simulink model "time_syn"  (R2016a)
settings: Solver=VariableStepAuto  StartTime=0.0  StopTime=1  RelTol=1e-3
values from neighbouring files (symbols this model uses):
  snr = SNR(i)    [mplot.m]
libraries: commchan3 x2, commdigbbndpm3 x1, commrandsrc2 x1, simulink x1, dspobslib x1, dspxfrm3 x1
settings Model: Creator=dell  LastModifiedBy=dell

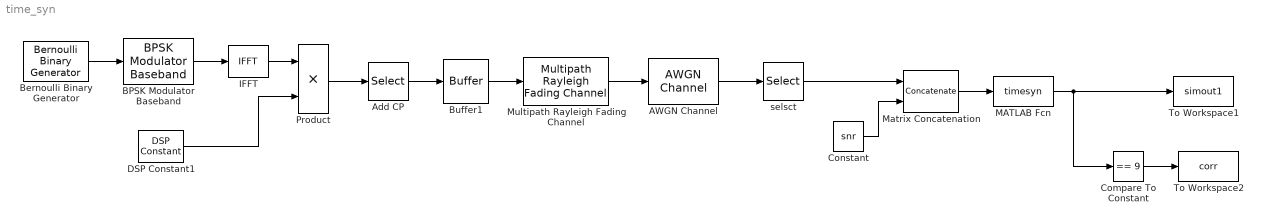
== system time_syn ==
  AWGN Channel : commchan3/AWGN Channel  InputProcessing=Inherited (this choice will be removed - see release notes)  seed=67  noiseMode="Signal to noise ratio  (SNR)"  EbNodB=ebn0  EsNodB=10  SNRdB=snr  bitsPerSym=1  Ps=1  Tsym=1/480000  variance=1
  Add CP : Selector  InputPortWidth=128  IndexOptions=Index vector (dialog)  Indices=[100:128 1:128]  OutputSizes=1
  BPSK Modulator Baseband : commdigbbndpm3/BPSK Modulator Baseband  Ph=0  outDtype=double  outWordLen=16  outUDDataType=sfix(16)  outFracLenMode=Best precision  outFracLen=15  outDataTypeStr=double  outLastDataTypeStr=double
  Bernoulli Binary Generator : commrandsrc2/Bernoulli Binary Generator  P=0.5  seed=565  Ts=1/480000  frameBased=on  sampPerFrame=128  orient=off  outDataType=double
  Buffer1 : Buffer  N=471
  Compare To Constant : simulink/Logic and Bit Operations/Compare To Constant  relop===  const=9  OutDataTypeStr=uint8  ZeroCross=off
  Constant : Constant  Value=snr
  DSP Constant1 : dspobslib/DSP Constant  Value=sqrt(128)  SampleMode=Discrete  discreteOutput=Sample-based  continuousOutput=Sample-based  sampTime=inf  framePeriod=2  dataType=Inherit from 'Constant value'  isSigned=on  wordLen=16  udDataType=sfix(16)  fracBitsMode=Best precision  numFracBits=15  InterpretAs1D=-inf  Ts=-inf  FramebasedOutput=-inf
  IFFT : dspxfrm3/IFFT  FFTImplementation=Auto  CompMethod=Table lookup  TableOpt=HYBRID  TableOptActive=Speed  BitRevOrder=off  cs_in=off  Normalize=on  InheritFFTLength=on  FFTLength=64  WrapInput=on  mode=Complex  outSamplingMode=Frame based  roundingMode=Floor  overflowMode=off  firstCoeffDataTypeStr=Inherit: Same word length as input  firstCoeffLastDataTypeStr=Inherit: Same word length as input  outputMin=[]  outputMax=[]
  MATLAB Fcn : MATLABFcn  MATLABFcn=timesyn  Output1D=off
  Matrix Concatenation : Concatenate  Mode=Multidimensional array
  Multipath Rayleigh Fading Channel : commchan3/Multipath Rayleigh Fading Channel  maxDopplerShift=40  spectrumType=Jakes  sigmaGaussian=1/sqrt(2)  coeffRounded=[1 -1.72 0.785]  freqMinMaxRJakes=[0 1]  freqMinMaxAJakes=[0 1]  sigmaGaussian1=1/sqrt(2)  sigmaGaussian2=1/sqrt(2)  centerFreqGaussian1=0.0  centerFreqGaussian2=0.0  gainGaussian1=0.5  gainGaussian2=0.5  coeffBell=9  dopplerSpectrum=doppler.jakes  pathDelays=[0 ]  avgPathGaindB=[0 ]  normalizePathGains=on  seed=73  enableProbe=0  openVisAtStart=off  outPathGains=off  outDelay=off
  Product : Product  RndMeth=Zero
  To Workspace1 : ToWorkspace  VariableName=simout1  SampleTime=-1
      settings: Save2DSignal=2-D array (concatenate along first dimension)
  To Workspace2 : ToWorkspace  VariableName=corr  SampleTime=-1
      settings: Save2DSignal=2-D array (concatenate along first dimension)
  selsct : Selector  InputPortWidth=471  IndexOptions=Index vector (dialog)  Indices=[150:335]  OutputSizes=1
  wires:
  IFFT/1 -> Product/1
  DSP Constant1/1 -> Product/2
  Product/1 -> Add CP/1
  BPSK Modulator Baseband/1 -> IFFT/1
  Add CP/1 -> Buffer1/1
  Buffer1/1 -> Multipath Rayleigh Fading Channel/1
  MATLAB Fcn/1 -> To Workspace1/1, Compare To Constant/1
  AWGN Channel/1 -> selsct/1
  Multipath Rayleigh Fading Channel/1 -> AWGN Channel/1
  selsct/1 -> Matrix Concatenation/1
  Constant/1 -> Matrix Concatenation/2
  Matrix Concatenation/1 -> MATLAB Fcn/1
  Compare To Constant/1 -> To Workspace2/1
  Bernoulli Binary Generator/1 -> BPSK Modulator Baseband/1
